simulink model "OLRippleTest"  (R2024a)
settings: Solver=VariableStepAuto  StartTime=0.0  StopTime=0.01  MaxStep=1e-6  RelTol=1e-3
undefined symbols (not defined in the file or in its folder): fs
libraries: cstblocks x4
settings Model: Creator=FactCore  LastModifiedBy=FactCore

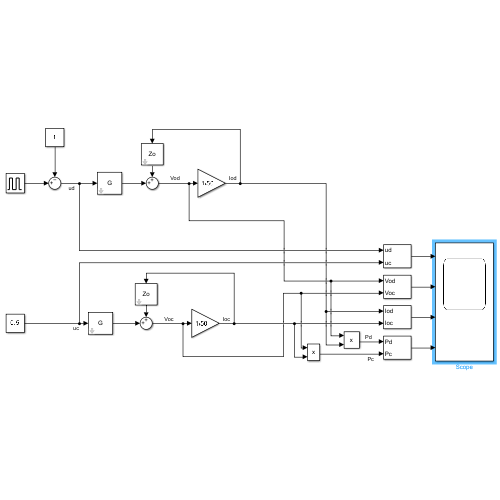
[thumbnail: Simulink's stored preview of the top-level diagram]
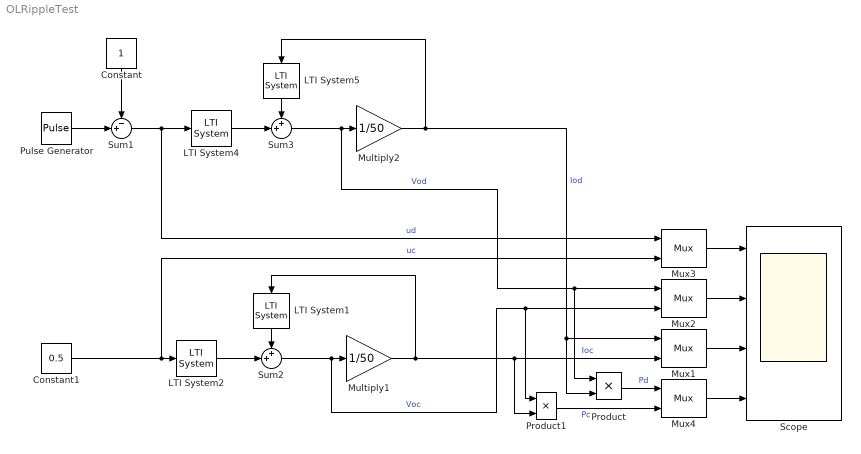
== system OLRippleTest ==
  Constant : Constant
  Constant1 : Constant  Value=0.5
  LTI System1 : cstblocks/LTI System  sys=Zo  IC=[]  PadeOrder=0
  LTI System2 : cstblocks/LTI System  sys=G  IC=[]  PadeOrder=0
  LTI System4 : cstblocks/LTI System  sys=G  IC=[]  PadeOrder=0
  LTI System5 : cstblocks/LTI System  sys=Zo  IC=[]  PadeOrder=0
  Multiply1 : Gain  Gain=1/50
  Multiply2 : Gain  Gain=1/50
  Mux{1..4} (4 alike) : Mux  Inputs=2
      settings: DisplayOption=signals
  Product : Product
  Product1 : Product
  Pulse Generator : DiscretePulseGenerator  PulseType=Time based  Amplitude=2  Period=1/fs  PulseWidth=75
  Scope : Scope  NumInputPorts=4
  Sum1 : Sum  Inputs=-+|
  Sum2 : Sum  Inputs=++|
  Sum3 : Sum  Inputs=++|
  wires:
  Multiply2/1 -> Product/2, Mux1/1, LTI System5/1  "Iod"
  Pulse Generator/1 -> Sum1/2
  Sum1/1 -> Mux3/1, LTI System4/1  "ud"
  Constant/1 -> Sum1/1
  Constant1/1 -> Mux3/2, LTI System2/1  "uc"
  Multiply1/1 -> Product1/2, Mux1/2, LTI System1/1  "Ioc"
  Mux3/1 -> Scope/1
  Mux1/1 -> Scope/3
  Mux2/1 -> Scope/2
  Mux4/1 -> Scope/4
  Product1/1 -> Mux4/2  "Pc"
  Product/1 -> Mux4/1  "Pd"
  Sum3/1 -> Mux2/1, Product/1, Multiply2/1  "Vod"
  LTI System5/1 -> Sum3/1
  LTI System4/1 -> Sum3/2
  LTI System1/1 -> Sum2/1
  LTI System2/1 -> Sum2/2
  Sum2/1 -> Product1/1, Mux2/2, Multiply1/1  "Voc"
